simulink model "xt2_1"  (R2014a)
settings: Solver=ode45  StartTime=0.0  StopTime=50  MaxStep=0.1  RelTol=1e-3
settings Model: Creator=tzb  LastModifiedBy=tzb
settings DebuggingCC: SolverPrmCheckMsg=none

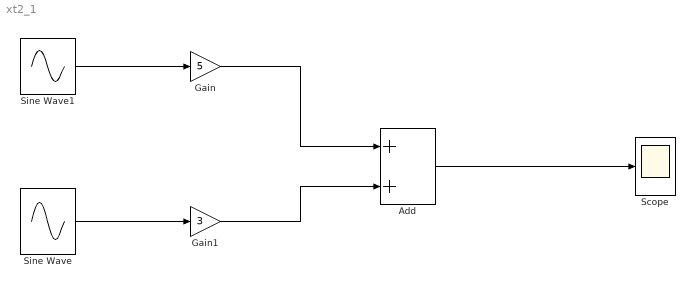
== system xt2_1 ==
  Add : Sum
  Gain : Gain  Gain=5
  Gain1 : Gain  Gain=3
  Scope : Scope
  Sine Wave : Sin  Frequency=2  SampleTime=0
  Sine Wave1 : Sin  Phase=pi/2  SampleTime=0
  wires:
  Add/1 -> Scope/1
  Sine Wave1/1 -> Gain/1
  Gain/1 -> Add/1
  Sine Wave/1 -> Gain1/1
  Gain1/1 -> Add/2
